simulink model "UGRP_Drone_Modeling4_with_motor_dynamics_v2_current_model"  (R2021b)
settings: Solver=FixedStepAuto  StartTime=0.0  StopTime=27  FixedStep=1/600
undefined symbols (not defined in the file or in its folder): sigbuilder_block
libraries: sim3dlib x1, uavsim3dlib x1
settings Model: Creator=user  LastModifiedBy=user
settings SolverCC: MaxConsecutiveMinStep=5  ShapePreserveControl=EnableAll  ZeroCrossAlgorithm=Adaptive
settings DebuggingCC: MaskedZcDiagnostic=none  IgnoredZcDiagnostic=none
settings SFSimCC: SimHardwareAcceleration=native  SimTargetLang=C++

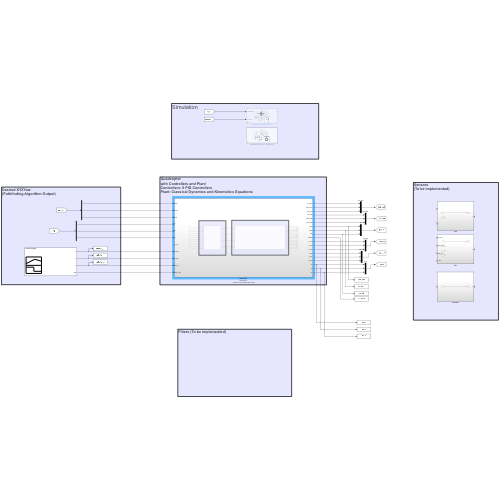
[thumbnail: Simulink's stored preview of the top-level diagram]
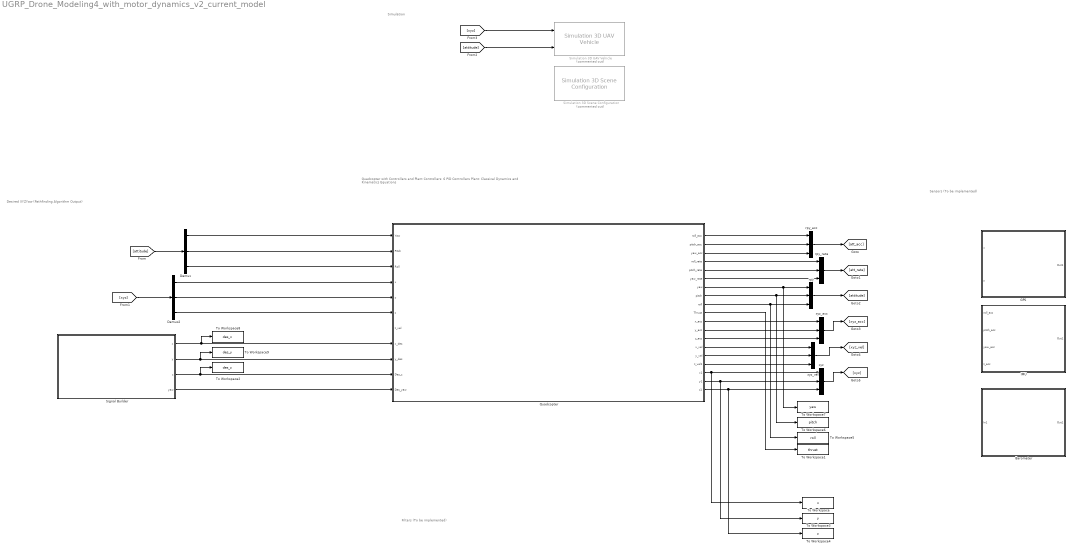
== system UGRP_Drone_Modeling4_with_motor_dynamics_v2_current_model ==
  note: Filters (To be implemented)
  note: Sensors
      | (To be implemented)
  note: Desired XYZYaw
      | (Pathfinding Algorithm Output)
  note: Quadcopter
      | with Controllers and Plant
      | Controllers: 6 PID Controllers
      | Plant: Classical Dynamics and Kinematics Equations
  note: Simulation
  Barometer : Subsystem
  Demux : Demux  Outputs=3
  Demux2 : Demux  Outputs=3
  GPS : Subsystem
  IMU : Subsystem
  Quadcopter : Subsystem  Description=Quadcopter including controllers and plant
      settings: AttributesFormatString=|
      | Quadcopter
      | - Controller and Quadcopter Plant
  Signal Builder : Subsystem  Tag=STV Subsys  LoadFcn=sigbuilder_block('load');  StartFcn=sigbuilder_block('start');  StopFcn=sigbuilder_block('stop');  ClipboardFcn=sigbuilder_block('clipboard');  mask(Sigbuilder block){tuvar=[0:10]}
      mask help: Simulink:masks:SigbuilderBlock_MD
      mask init:
      | if ~strcmp(get_param(bdroot(gcbh),'SimulationStatus'),'stopped') tuvar = sigbuilder_block('maskInit'); end
      settings: CopyFcn=sigbuilder_block('copy');  DeleteFcn=sigbuilder_block('delete');  ModelCloseFcn=sigbuilder_block('modelClose');  PreSaveFcn=sigbuilder_block('preSave');  PauseFcn=sigbuilder_block('pause');  ContinueFcn=sigbuilder_block('continue');  NameChangeFcn=sigbuilder_block('namechange');  OpenFcn=sigbuilder_block('open',[304.5 213 821.25 385.5 ]);  CloseFcn=sigbuilder_block('close');
      mask Display: plot(0, 0, 100, 100,[2, 2, 32, 32, 2], [68, 8, 8, 68, 68],[32, 2], [38, 38], [32, 19, 2],[53, 60, 44], [32, 17, 17, 2],[16, 16, 31, 31]);txt = getActiveGroup(gcbh);text(2, 100, txt,'verticalAlignment', 'top');
  Simulation 3D Scene Configuration : sim3dlib/Simulation 3D Scene Configuration  Priority=0  Commented=on  ProjectFormat_internal=Default Scenes  ProjectFormat=Default Scenes  SceneDesc=US city block  ProjectName=C:\Program Files\MATLAB\R2021b\toolbox\shared\sim3d_projects\automotive_project\UE4\WindowsNoEditor\VehicleSimulation.exe  ScenePath=/Game/Maps/USCityBlock  vehTagList={'Scene Origin';'SimulinkVehicle1'}  vehTag=SimulinkVehicle1  OpVisEn=off  Ts=1/60  EnableWindow=on  EnableWeather=off  SunAltitude=40.0  SunAzimuth=90  clouds=10  wind=1  fog=0  rain=0  sensorTag=MainCamera1  sensorId=1  sensorName=MainCamera1  mountLoc=Origin  offsetFlag=off  tmountOffset=[0, 0, 0]  rmountOffset=[0, 0, 0]  HorizontalResolution=1280  VerticalResolution=720  HorizontalFOV=60  mountPoint=[0 0 0]  mountOrientation=[0 0 0]  aMode=4  ID=1
      settings: SourceProductBaseCode=AE,DR,UV,VE
  Simulation 3D UAV Vehicle : uavsim3dlib/Simulation 3D UAV Vehicle  Priority=-1  Commented=on  Mesh=Quadrotor  MeshPath=/MathWorksUAVContent/UAVs/HexaRotorUAV/HexaRotor.HexaRotor  Color=Black  ActorName=SimulinkVehicle1  InitialTranslation=[0 0 0]  InitialRotation=[0 0 0]  SampleTime=-1  ActorType=SimulinkVehicle  ID=1  aMode=4  ActorTag=SimulinkVehicle1
      settings: SourceProductBaseCode=UV
  To Workspace : ToWorkspace  VariableName=x  SaveFormat=Timeseries  SampleTime=-1
  To Workspace1 : ToWorkspace  VariableName=thrust  SaveFormat=Timeseries  SampleTime=-1
  To Workspace2 : ToWorkspace  VariableName=des_z  SaveFormat=Timeseries  SampleTime=-1
  To Workspace3 : ToWorkspace  VariableName=y  SaveFormat=Timeseries  SampleTime=-1
  To Workspace4 : ToWorkspace  VariableName=z  SaveFormat=Timeseries  SampleTime=-1
  To Workspace5 : ToWorkspace  VariableName=roll  SaveFormat=Timeseries  SampleTime=-1
  To Workspace6 : ToWorkspace  VariableName=pitch  SaveFormat=Timeseries  SampleTime=-1
  To Workspace7 : ToWorkspace  VariableName=yaw  SaveFormat=Timeseries  SampleTime=-1
  To Workspace8 : ToWorkspace  VariableName=des_x  SaveFormat=Timeseries  SampleTime=-1
  To Workspace9 : ToWorkspace  VariableName=des_y  SaveFormat=Timeseries  SampleTime=-1
  rpy : Mux  Inputs=3
  rpy_acc : Mux  Inputs=3
  rpy_rate : Mux  Inputs=3
  xyz : Mux  Inputs=3
  xyz_acc : Mux  Inputs=3
  xyz_vel : Mux  Inputs=3
  wires:
  Signal Builder/3(z) -> Quadcopter/10(Des_z), To Workspace2/1
  xyz/1 -> [xyz]
  rpy/1 -> [attitude]
  rpy_acc/1 -> [att_acc]
  rpy_rate/1 -> [att_rate]
  xyz_acc/1 -> [xyz_acc]
  xyz_vel/1 -> [xyz_vel]
  [xyz] -> Demux2/1
  [attitude] -> Demux/1
  Quadcopter/7(yaw) -> rpy/1, To Workspace7/1
  Quadcopter/9(roll) -> rpy/3, To Workspace5/1
  Quadcopter/8(pitch) -> To Workspace6/1, rpy/2
  Demux/1 -> Quadcopter/1(Yaw)
  Demux/2 -> Quadcopter/2(Pitch)
  Demux/3 -> Quadcopter/3(Roll)
  Demux2/1 -> Quadcopter/4(x)
  Demux2/2 -> Quadcopter/5(y)
  Demux2/3 -> Quadcopter/6(z)
  Signal Builder/4(yaw) -> Quadcopter/11(Des_yaw)
  Quadcopter/1(roll_acc) -> rpy_acc/1
  Quadcopter/2(pitch_acc) -> rpy_acc/2
  Quadcopter/3(yaw_acc) -> rpy_acc/3
  Quadcopter/4(roll_rate) -> rpy_rate/1
  Quadcopter/5(pitch_rate) -> rpy_rate/2
  Quadcopter/6(yaw_rate) -> rpy_rate/3
  Quadcopter/11(x_acc) -> xyz_acc/1
  Quadcopter/12(y_acc) -> xyz_acc/2
  Quadcopter/13(z_acc) -> xyz_acc/3
  Quadcopter/14(x_vel) -> xyz_vel/1
  Quadcopter/15(y_vel) -> xyz_vel/2
  Quadcopter/16(z_vel1) -> xyz_vel/3
  Quadcopter/17(x1) -> xyz/1, To Workspace/1
  Quadcopter/18(y1) -> xyz/2, To Workspace3/1
  Quadcopter/19(z1) -> xyz/3, To Workspace4/1
  Quadcopter/10(Thrust) -> To Workspace1/1
  [xyz] -> Simulation 3D UAV Vehicle/1
  [attitude] -> Simulation 3D UAV Vehicle/2
  Signal Builder/1(x) -> Quadcopter/8(x_des), To Workspace8/1
  Signal Builder/2(y) -> Quadcopter/9(y_des), To Workspace9/1

== system UGRP_Drone_Modeling4_with_motor_dynamics_v2_current_model/Barometer ==
  In1 : Inport
  Out1 : Outport
  wires:
  In1/1 -> Out1/1

== system UGRP_Drone_Modeling4_with_motor_dynamics_v2_current_model/GPS ==
  x : Inport
  y : Inport  Port=2
  Out1 : Outport
  wires:
  x/1 -> Out1/1

== system UGRP_Drone_Modeling4_with_motor_dynamics_v2_current_model/IMU ==
  roll_acc : Inport
  pitch_acc : Inport  Port=2
  yaw_acc : Inport  Port=3
  z_acc : Inport  Port=4
  Out1 : Outport
  wires:
  roll_acc/1 -> Out1/1

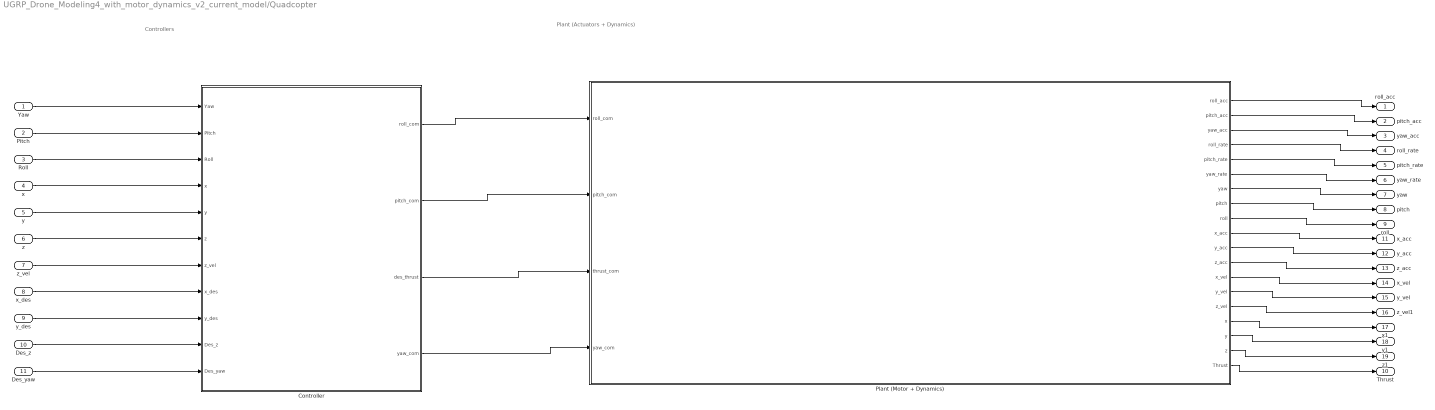
== system UGRP_Drone_Modeling4_with_motor_dynamics_v2_current_model/Quadcopter ==
  note: Plant (Actuators + Dynamics)
  note: Controllers
  Yaw : Inport
  Pitch : Inport  Port=2
  Roll : Inport  Port=3
  x : Inport  Port=4
  y : Inport  Port=5
  z : Inport  Port=6
  z_vel : Inport  Port=7
  x_des : Inport  Port=8
  y_des : Inport  Port=9
  Des_z : Inport  Port=10
  Des_yaw : Inport  Port=11
  Controller : Subsystem
  Plant (Motor + Dynamics) : Subsystem
  roll_acc : Outport
  pitch_acc : Outport  Port=2
  yaw_acc : Outport  Port=3
  roll_rate : Outport  Port=4
  pitch_rate : Outport  Port=5
  yaw_rate : Outport  Port=6
  yaw : Outport  Port=7
  pitch : Outport  Port=8
  roll : Outport  Port=9
  Thrust : Outport  Port=10
  x_acc : Outport  Port=11
  y_acc : Outport  Port=12
  z_acc : Outport  Port=13
  x_vel : Outport  Port=14
  y_vel : Outport  Port=15
  z_vel1 : Outport  Port=16
  x1 : Outport  Port=17
  y1 : Outport  Port=18
  z1 : Outport  Port=19
  wires:
  Plant (Motor + Dynamics)/14(y_vel) -> y_vel/1
  Plant (Motor + Dynamics)/9(roll) -> roll/1
  x_des/1 -> Controller/8(x_des)
  Controller/1(roll_com) -> Plant (Motor + Dynamics)/1(roll_com)
  Plant (Motor + Dynamics)/6(yaw_rate) -> yaw_rate/1
  Plant (Motor + Dynamics)/7(yaw) -> yaw/1
  Plant (Motor + Dynamics)/17(y) -> y1/1
  Plant (Motor + Dynamics)/18(z) -> z1/1
  Controller/2(pitch_com) -> Plant (Motor + Dynamics)/2(pitch_com)
  Plant (Motor + Dynamics)/5(pitch_rate) -> pitch_rate/1
  Plant (Motor + Dynamics)/10(x_acc) -> x_acc/1
  Des_yaw/1 -> Controller/11(Des_yaw)
  Controller/3(des_thrust) -> Plant (Motor + Dynamics)/3(thrust_com)
  Plant (Motor + Dynamics)/8(pitch) -> pitch/1
  Controller/4(yaw_com) -> Plant (Motor + Dynamics)/4(yaw_com)
  Plant (Motor + Dynamics)/13(x_vel) -> x_vel/1
  y/1 -> Controller/5(y)
  Plant (Motor + Dynamics)/1(roll_acc) -> roll_acc/1
  Des_z/1 -> Controller/10(Des_z)
  Plant (Motor + Dynamics)/19(Thrust) -> Thrust/1
  x/1 -> Controller/4(x)
  Plant (Motor + Dynamics)/3(yaw_acc) -> yaw_acc/1
  Plant (Motor + Dynamics)/12(z_acc) -> z_acc/1
  Plant (Motor + Dynamics)/11(y_acc) -> y_acc/1
  Roll/1 -> Controller/3(Roll)
  Plant (Motor + Dynamics)/15(z_vel) -> z_vel1/1
  z_vel/1 -> Controller/7(z_vel)
  Plant (Motor + Dynamics)/16(x) -> x1/1
  y_des/1 -> Controller/9(y_des)
  Yaw/1 -> Controller/1(Yaw)
  Plant (Motor + Dynamics)/2(pitch_acc) -> pitch_acc/1
  z/1 -> Controller/6(z)
  Pitch/1 -> Controller/2(Pitch)
  Plant (Motor + Dynamics)/4(roll_rate) -> roll_rate/1

== system UGRP_Drone_Modeling4_with_motor_dynamics_v2_current_model/Signal Builder ==
  Demux : Demux  Tag=STV Demux
      settings: DisplayOption=none
  FromWs : FromWorkspace  Tag=STV FromWs  VariableName=tuvar
      SigBuilderData=|
      | common.afterFinalStr = 'Extrapolate'
      | common.sampleTime = 0
      | dataSet.timeRange = [0 25]
      | dataSet.name = 'Desired xyzyaw'
      | sbobj.Groups.Name = 'Desired xyzyaw'
      | sbobj.Groups.Signals(1).Name = 'x'
      | sbobj.Groups.Signals(1).XData = [0 12 12 20 20 25]
      | sbobj.Groups.Signals(1).YData = [0 0 2 2 0 0]
      | sbobj.Groups.Signals(2).Name = 'y'
      | sbobj.Groups.Signals(2).XData = [0 3.99 12 12 20 20 25]
      | sbobj.Groups.Signals(2).YData = [0 0 0 -2 -2 0 0]
      | sbobj.Groups.Signals(3).Name = 'z'
      | sbobj.Groups.Signals(3).XData = [0 25]
      | sbobj.Groups.Signals(3).YData = [3 3]
      | sbobj.Groups.Signals(4).Name = 'yaw'
      | sbobj.Groups.Signals(4).XData = [0 5 8 25]
      | sbobj.Groups.Signals(4).YData = [0 0 0 0]
      | sbobj.Groups.TimeRange = [0 25]
  x : Outport  Tag=STV Outport
  y : Outport  Tag=STV Outport  Port=2
  z : Outport  Tag=STV Outport  Port=3
  yaw : Outport  Tag=STV Outport  Port=4
  wires:
  FromWs/1 -> Demux/1
  Demux/1 -> x/1
  Demux/2 -> y/1
  Demux/3 -> z/1
  Demux/4 -> yaw/1

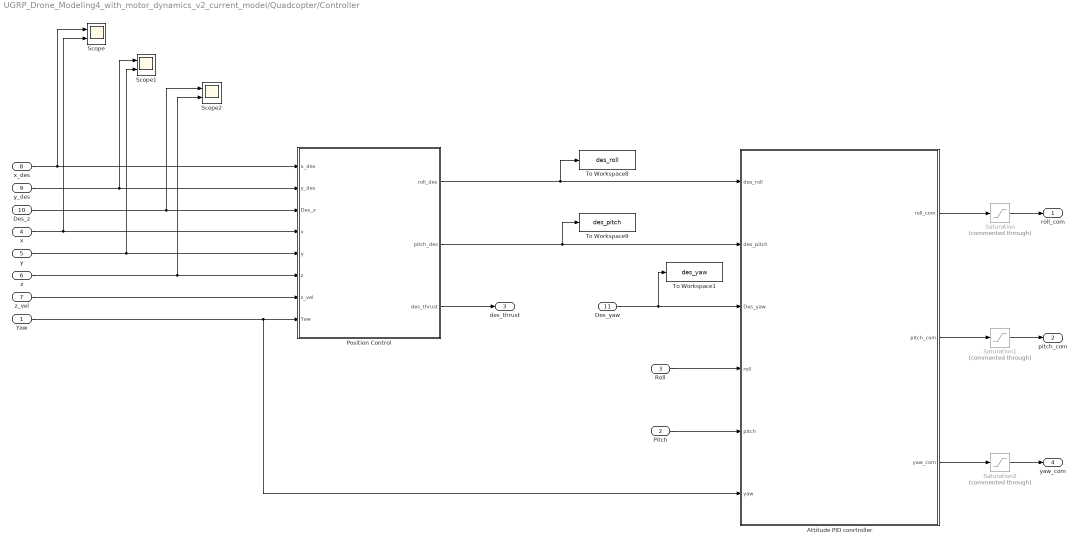
== system UGRP_Drone_Modeling4_with_motor_dynamics_v2_current_model/Quadcopter/Controller ==
  Yaw : Inport
  Pitch : Inport  Port=2
  Roll : Inport  Port=3
  x : Inport  Port=4
  y : Inport  Port=5
  z : Inport  Port=6
  z_vel : Inport  Port=7
  x_des : Inport  Port=8
  y_des : Inport  Port=9
  Des_z : Inport  Port=10
  Des_yaw : Inport  Port=11
  Attitude PID conrtroller : Subsystem
  Position Control : Subsystem
  Saturation : Saturate  Commented=through  UpperLimit=4  LowerLimit=-4
  Saturation1 : Saturate  Commented=through  UpperLimit=1  LowerLimit=-1
  Saturation2 : Saturate  Commented=through  UpperLimit=1  LowerLimit=-1
  Scope : Scope  NumInputPorts=2
  Scope1 : Scope  NumInputPorts=2
  Scope2 : Scope  NumInputPorts=2
  To Workspace1 : ToWorkspace  VariableName=des_yaw  SaveFormat=Timeseries  SampleTime=-1
  To Workspace8 : ToWorkspace  VariableName=des_roll  SaveFormat=Timeseries  SampleTime=-1
  To Workspace9 : ToWorkspace  VariableName=des_pitch  SaveFormat=Timeseries  SampleTime=-1
  roll_com : Outport
  pitch_com : Outport  Port=2
  des_thrust : Outport  Port=3
  yaw_com : Outport  Port=4
  wires:
  z_vel/1 -> Position Control/7(z_vel)
  Attitude PID conrtroller/2(pitch_com) -> Saturation1/1
  Position Control/3(des_thrust) -> des_thrust/1
  y/1 -> Scope1/2, Position Control/5(y)
  Attitude PID conrtroller/3(yaw_com) -> Saturation2/1
  Attitude PID conrtroller/1(roll_com) -> Saturation/1
  Des_yaw/1 -> Attitude PID conrtroller/3(Des_yaw), To Workspace1/1
  x_des/1 -> Position Control/1(x_des), Scope/1
  z/1 -> Position Control/6(z), Scope2/2
  Des_z/1 -> Position Control/3(Des_z), Scope2/1
  y_des/1 -> Scope1/1, Position Control/2(y_des)
  Yaw/1 -> Attitude PID conrtroller/6(yaw), Position Control/8(Yaw)
  x/1 -> Position Control/4(x), Scope/2
  Position Control/2(pitch_des) -> To Workspace9/1, Attitude PID conrtroller/2(des_pitch)
  Position Control/1(roll_des) -> To Workspace8/1, Attitude PID conrtroller/1(des_roll)
  Roll/1 -> Attitude PID conrtroller/4(roll)
  Pitch/1 -> Attitude PID conrtroller/5(pitch)
  Saturation/1 -> roll_com/1
  Saturation1/1 -> pitch_com/1
  Saturation2/1 -> yaw_com/1

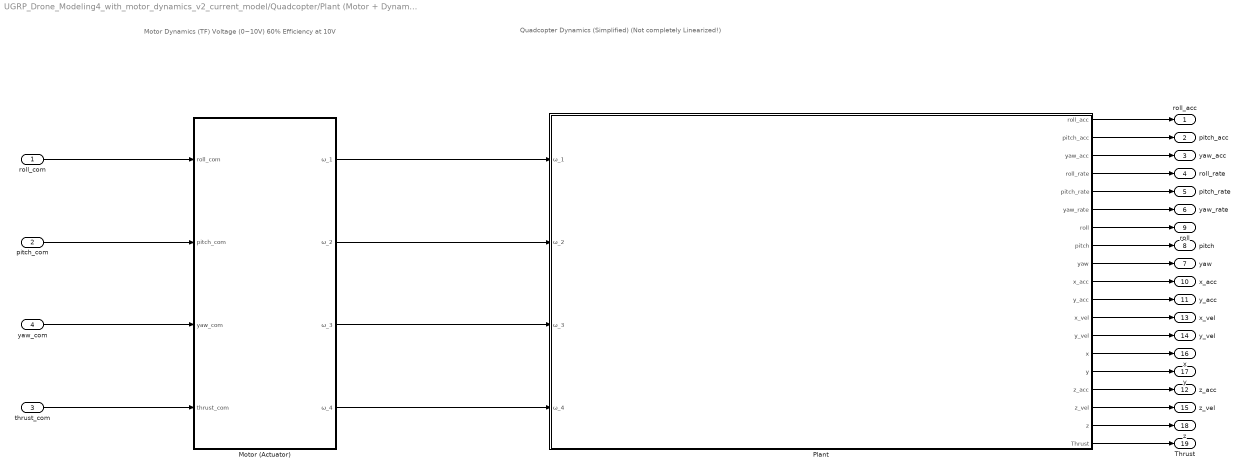
== system UGRP_Drone_Modeling4_with_motor_dynamics_v2_current_model/Quadcopter/Plant (Motor + Dynamics) ==
  note: Quadcopter Dynamics  (Simplified)
      | (Not completely Linearized!)
  note: Motor Dynamics (TF)
      | Voltage (0~10V)
      | 60% Efficiency at 10V
  roll_com : Inport
  pitch_com : Inport  Port=2
  thrust_com : Inport  Port=3
  yaw_com : Inport  Port=4
  Motor (Actuator) : Subsystem
  Plant : Subsystem
  roll_acc : Outport
  pitch_acc : Outport  Port=2
  yaw_acc : Outport  Port=3
  roll_rate : Outport  Port=4
  pitch_rate : Outport  Port=5
  yaw_rate : Outport  Port=6
  yaw : Outport  Port=7
  pitch : Outport  Port=8
  roll : Outport  Port=9
  x_acc : Outport  Port=10
  y_acc : Outport  Port=11
  z_acc : Outport  Port=12
  x_vel : Outport  Port=13
  y_vel : Outport  Port=14
  z_vel : Outport  Port=15
  x : Outport  Port=16
  y : Outport  Port=17
  z : Outport  Port=18
  Thrust : Outport  Port=19
  wires:
  Plant/9(yaw) -> yaw/1
  Motor (Actuator)/1(ω_1) -> Plant/1(ω_1)
  Plant/2(pitch_acc) -> pitch_acc/1
  Motor (Actuator)/2(ω_2) -> Plant/2(ω_2)
  Plant/7(roll) -> roll/1
  Motor (Actuator)/4(ω_4) -> Plant/4(ω_4)
  Plant/6(yaw_rate) -> yaw_rate/1
  Plant/8(pitch) -> pitch/1
  Plant/5(pitch_rate) -> pitch_rate/1
  Motor (Actuator)/3(ω_3) -> Plant/3(ω_3)
  Plant/12(x_vel) -> x_vel/1
  Plant/11(y_acc) -> y_acc/1
  Plant/13(y_vel) -> y_vel/1
  Plant/4(roll_rate) -> roll_rate/1
  Plant/1(roll_acc) -> roll_acc/1
  roll_com/1 -> Motor (Actuator)/1(roll_com)
  Plant/3(yaw_acc) -> yaw_acc/1
  Plant/10(x_acc) -> x_acc/1
  pitch_com/1 -> Motor (Actuator)/2(pitch_com)
  Plant/14(x) -> x/1
  Plant/16(z_acc) -> z_acc/1
  Plant/19(Thrust) -> Thrust/1
  Plant/15(y) -> y/1
  Plant/17(z_vel) -> z_vel/1
  Plant/18(z) -> z/1
  yaw_com/1 -> Motor (Actuator)/3(yaw_com)
  thrust_com/1 -> Motor (Actuator)/4(thrust_com)

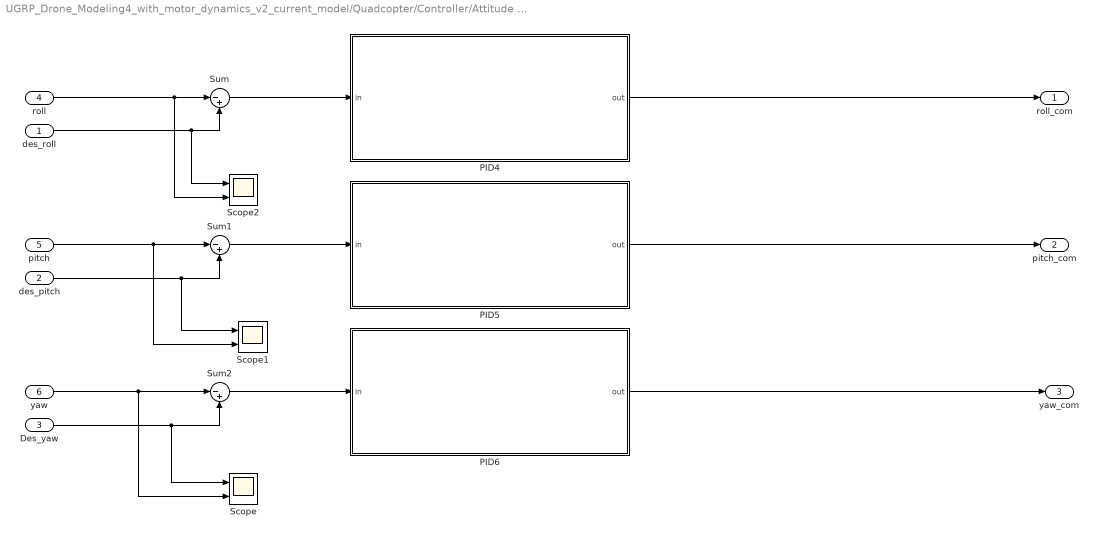
== system UGRP_Drone_Modeling4_with_motor_dynamics_v2_current_model/Quadcopter/Controller/Attitude PID conrtroller ==
  des_roll : Inport
  des_pitch : Inport  Port=2
  Des_yaw : Inport  Port=3
  roll : Inport  Port=4
  pitch : Inport  Port=5
  yaw : Inport  Port=6
  PID4 : Subsystem
  PID5 : Subsystem
  PID6 : Subsystem
  Scope : Scope  NumInputPorts=2
  Scope1 : Scope  NumInputPorts=2
  Scope2 : Scope  NumInputPorts=2
  Sum : Sum  Inputs=|-+
  Sum1 : Sum  Inputs=|-+
  Sum2 : Sum  Inputs=|-+
  roll_com : Outport
  pitch_com : Outport  Port=2
  yaw_com : Outport  Port=3
  wires:
  des_roll/1 -> Scope2/1, Sum/2
  Des_yaw/1 -> Scope/1, Sum2/2
  yaw/1 -> Scope/2, Sum2/1
  Sum/1 -> PID4/1(in)
  Sum2/1 -> PID6/1(in)
  Sum1/1 -> PID5/1(in)
  pitch/1 -> Scope1/2, Sum1/1
  des_pitch/1 -> Scope1/1, Sum1/2
  roll/1 -> Scope2/2, Sum/1
  PID4/1(out) -> roll_com/1
  PID5/1(out) -> pitch_com/1
  PID6/1(out) -> yaw_com/1

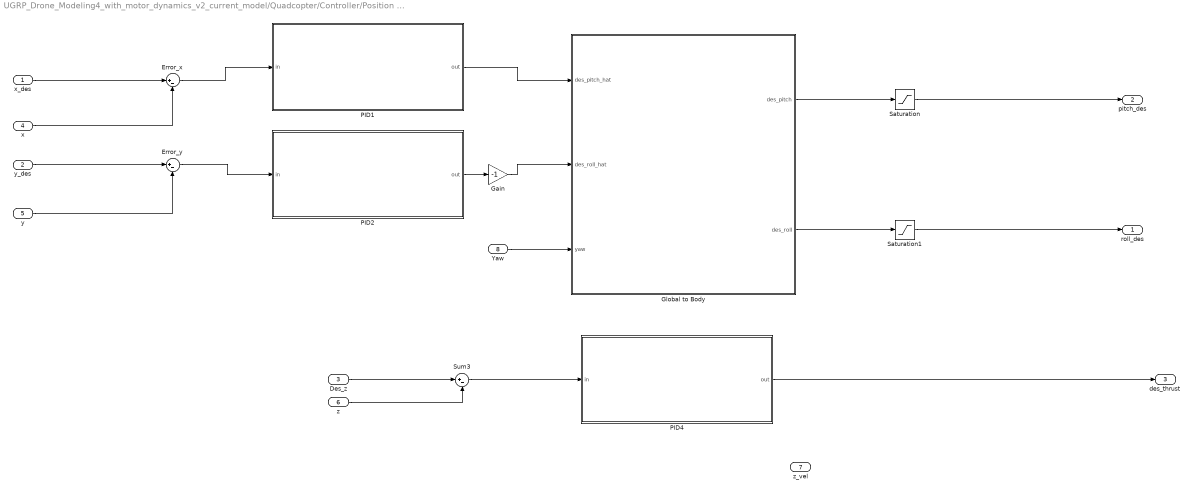
== system UGRP_Drone_Modeling4_with_motor_dynamics_v2_current_model/Quadcopter/Controller/Position Control ==
  x_des : Inport
  y_des : Inport  Port=2
  Des_z : Inport  Port=3
  x : Inport  Port=4
  y : Inport  Port=5
  z : Inport  Port=6
  z_vel : Inport  Port=7
  Yaw : Inport  Port=8
  Error_x : Sum  Inputs=|+-
  Error_y : Sum  Inputs=|+-
  Gain : Gain  Gain=-1
  Global to Body : Subsystem
  PID1 : Subsystem
  PID2 : Subsystem
  PID4 : Subsystem
  Saturation : Saturate  UpperLimit=10*pi/180  LowerLimit=-10*pi/180
  Saturation1 : Saturate  UpperLimit=10*pi/180  LowerLimit=-10*pi/180
  Sum3 : Sum  Inputs=|+-
  roll_des : Outport
  pitch_des : Outport  Port=2
  des_thrust : Outport  Port=3
  wires:
  x_des/1 -> Error_x/1
  x/1 -> Error_x/2
  y_des/1 -> Error_y/1
  y/1 -> Error_y/2
  Des_z/1 -> Sum3/1
  Yaw/1 -> Global to Body/3(yaw)
  Error_y/1 -> PID2/1(in)
  Error_x/1 -> PID1/1(in)
  Global to Body/2(des_roll) -> Saturation1/1
  z/1 -> Sum3/2
  Global to Body/1(des_pitch) -> Saturation/1
  PID1/1(out) -> Global to Body/1(des_pitch_hat)
  PID2/1(out) -> Gain/1
  Gain/1 -> Global to Body/2(des_roll_hat)
  Saturation1/1 -> roll_des/1
  Saturation/1 -> pitch_des/1
  Sum3/1 -> PID4/1(in)
  PID4/1(out) -> des_thrust/1

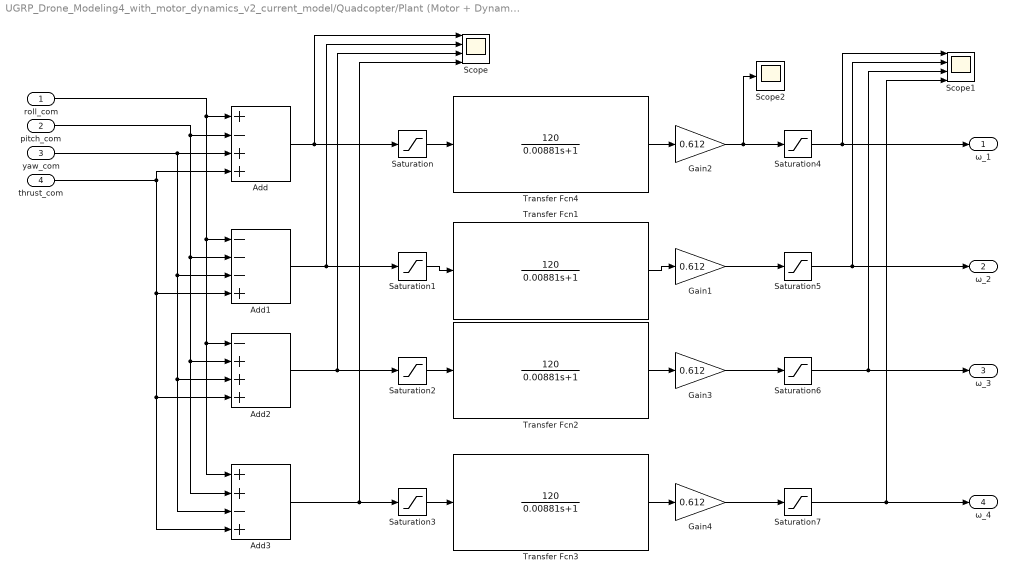
== system UGRP_Drone_Modeling4_with_motor_dynamics_v2_current_model/Quadcopter/Plant (Motor + Dynamics)/Motor (Actuator) ==
  roll_com : Inport
  pitch_com : Inport  Port=2
  yaw_com : Inport  Port=3
  thrust_com : Inport  Port=4
  Add : Sum  Inputs=+-++
  Add1 : Sum  Inputs=---+
  Add2 : Sum  Inputs=-+++
  Add3 : Sum  Inputs=++-+
  Gain{1..4} (4 alike) : Gain  Gain=0.612
  Saturation{,1..3} (4 alike) : Saturate  UpperLimit=10  LowerLimit=0
  Saturation{4..7} (4 alike) : Saturate  UpperLimit=1040  LowerLimit=0
  Scope : Scope  NumInputPorts=4
  Scope1 : Scope  NumInputPorts=4
  Scope2 : Scope
  Transfer Fcn{1..4} (4 alike) : TransferFcn  Numerator=[120]  Denominator=[0.00881 1]
  ω_1 : Outport
  ω_2 : Outport  Port=2
  ω_3 : Outport  Port=3
  ω_4 : Outport  Port=4
  wires:
  roll_com/1 -> Add3/1, Add2/1, Add1/1, Add/1
  pitch_com/1 -> Add3/2, Add2/2, Add1/2, Add/2
  yaw_com/1 -> Add3/3, Add2/3, Add1/3, Add/3
  thrust_com/1 -> Add/4, Add3/4, Add2/4, Add1/4
  Add/1 -> Saturation/1, Scope/1
  Add1/1 -> Saturation1/1, Scope/2
  Add2/1 -> Saturation2/1, Scope/3
  Add3/1 -> Scope/4, Saturation3/1
  Saturation/1 -> Transfer Fcn4/1
  Saturation2/1 -> Transfer Fcn2/1
  Saturation1/1 -> Transfer Fcn1/1
  Saturation3/1 -> Transfer Fcn3/1
  Saturation4/1 -> Scope1/1, ω_1/1
  Saturation5/1 -> Scope1/2, ω_2/1
  Saturation6/1 -> Scope1/3, ω_3/1
  Saturation7/1 -> Scope1/4, ω_4/1
  Transfer Fcn4/1 -> Gain2/1
  Gain2/1 -> Scope2/1, Saturation4/1
  Transfer Fcn1/1 -> Gain1/1
  Gain1/1 -> Saturation5/1
  Transfer Fcn2/1 -> Gain3/1
  Gain3/1 -> Saturation6/1
  Transfer Fcn3/1 -> Gain4/1
  Gain4/1 -> Saturation7/1

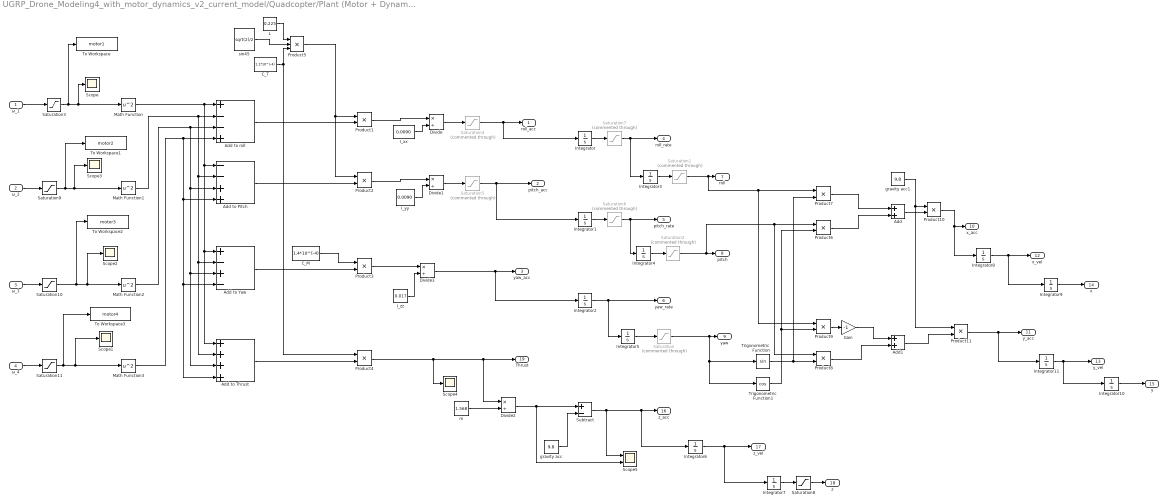
== system UGRP_Drone_Modeling4_with_motor_dynamics_v2_current_model/Quadcopter/Plant (Motor + Dynamics)/Plant ==
  ω_1 : Inport
  ω_2 : Inport  Port=2
  ω_3 : Inport  Port=3
  ω_4 : Inport  Port=4
  Add : Sum
  Add to Pitch : Sum  Inputs=--++  RndMeth=Round
  Add to Thrust : Sum  Inputs=++++  RndMeth=Round
  Add to Yaw : Sum  Inputs=+-+-  RndMeth=Round
  Add to roll : Sum  Inputs=+--+
  Add1 : Sum
  C_M : Constant  Value=1.4*10^(-4)
  C_T : Constant  Value=1.1*10^(-4)
  Divide{,1..3} (4 alike) : Product  Inputs=*/
  Gain : Gain  Gain=-1
  I_xx : Constant  Value=0.0090
  I_yy : Constant  Value=0.0090
  I_zz : Constant  Value=0.017
  Integrator{,1,6..11} (8 alike) : Integrator
  Integrator2 : Integrator  LimitOutput=on  UpperSaturationLimit=2*pi  LowerSaturationLimit=-2*pi  WrappedStateUpperValue=2*pi  WrappedStateLowerValue=-2*pi
  Integrator3 : Integrator  LimitOutput=on  UpperSaturationLimit=10*pi/180  LowerSaturationLimit=-10*pi/180  WrappedStateUpperValue=10*pi/180  WrappedStateLowerValue=-10*pi/180
  Integrator4 : Integrator  LimitOutput=on  UpperSaturationLimit=10*pi/180  LowerSaturationLimit=-10*pi/180  WrappedStateUpperValue=10*pi/180  WrappedStateLowerValue=-10*pi/180
  Integrator5 : Integrator  UpperSaturationLimit=pi  LowerSaturationLimit=-pi
  L : Constant  Value=0.225
  Math Function : Math  Operator=square  RndMeth=Round  SaturateOnIntegerOverflow=on
  Math Function1 : Math  Operator=square  SaturateOnIntegerOverflow=on
  Math Function2 : Math  Operator=square  SaturateOnIntegerOverflow=on
  Math Function3 : Math  Operator=square  SaturateOnIntegerOverflow=on
  Product{1..4,6..11} (10 alike) : Product
  Product5 : Product  Inputs=3
  Saturation : Saturate  Commented=through  UpperLimit=2*pi  LowerLimit=-2*pi
  Saturation1 : Saturate  Commented=through  UpperLimit=10*pi/180  LowerLimit=-10*pi/180
  Saturation{3,9..11} (4 alike) : Saturate  UpperLimit=1000  LowerLimit=0
  Saturation2 : Saturate  Commented=through  UpperLimit=10*pi/180  LowerLimit=-10*pi/180
  Saturation{4..7} (4 alike) : Saturate  Commented=through  UpperLimit=1  LowerLimit=-1
  Saturation8 : Saturate  UpperLimit=inf  LowerLimit=0
  Scope{,1..4} (5 alike) : Scope
  Scope5 : Scope  NumInputPorts=2
  Subtract : Sum  Inputs=+-
  To Workspace : ToWorkspace  VariableName=motor1  SaveFormat=Timeseries  SampleTime=-1
  To Workspace1 : ToWorkspace  VariableName=motor2  SaveFormat=Timeseries  SampleTime=-1
  To Workspace2 : ToWorkspace  VariableName=motor3  SaveFormat=Timeseries  SampleTime=-1
  To Workspace3 : ToWorkspace  VariableName=motor4  SaveFormat=Timeseries  SampleTime=-1
  Trigonometric Function : Trigonometry
  Trigonometric Function1 : Trigonometry  Operator=cos
  gravity acc : Constant  Value=9.8
  gravity acc1 : Constant  Value=9.8
  m : Constant  Value=1.568
  sin45 : Constant  Value=sqrt(2)/2
  roll_acc : Outport
  pitch_acc : Outport  Port=2
  yaw_acc : Outport  Port=3
  roll_rate : Outport  Port=4
  pitch_rate : Outport  Port=5
  yaw_rate : Outport  Port=6
  roll : Outport  Port=7
  pitch : Outport  Port=8
  yaw : Outport  Port=9
  x_acc : Outport  Port=10
  y_acc : Outport  Port=11
  x_vel : Outport  Port=12
  y_vel : Outport  Port=13
  x : Outport  Port=14
  y : Outport  Port=15
  z_acc : Outport  Port=16
  z_vel : Outport  Port=17
  z : Outport  Port=18
  Thrust : Outport  Port=19
  wires:
  Product5/1 -> Product2/1, Product1/1
  ω_1/1 -> Saturation3/1
  ω_3/1 -> Saturation10/1
  ω_4/1 -> Saturation11/1
  Math Function/1 -> Add to Thrust/1, Add to Yaw/1, Add to Pitch/1, Add to roll/1
  Math Function1/1 -> Add to Thrust/2, Add to Yaw/2, Add to Pitch/2, Add to roll/2
  Math Function2/1 -> Add to Thrust/3, Add to Yaw/3, Add to Pitch/3, Add to roll/3
  Math Function3/1 -> Add to Thrust/4, Add to Yaw/4, Add to Pitch/4, Add to roll/4
  Add to roll/1 -> Product1/2
  Add to Yaw/1 -> Product3/2
  Add to Thrust/1 -> Product4/2
  sin45/1 -> Product5/2
  L/1 -> Product5/1
  C_M/1 -> Product3/1
  Product1/1 -> Divide/1
  I_xx/1 -> Divide/2
  Product2/1 -> Divide1/1
  I_yy/1 -> Divide1/2
  Divide/1 -> Saturation4/1
  Integrator2/1 -> Integrator5/1, yaw_rate/1
  Integrator1/1 -> Saturation6/1
  Integrator/1 -> Saturation7/1
  m/1 -> Divide2/2
  gravity acc/1 -> Subtract/2
  Integrator4/1 -> Saturation2/1
  Integrator3/1 -> Saturation1/1
  Saturation1/1 -> Product9/1, Product7/1, roll/1
  Integrator6/1 -> Integrator7/1, z_vel/1
  Integrator7/1 -> Saturation8/1
  Integrator8/1 -> Integrator9/1, x_vel/1
  Integrator9/1 -> x/1
  Integrator10/1 -> y/1
  Integrator11/1 -> Integrator10/1, y_vel/1
  C_T/1 -> Product5/3, Product4/1
  Product3/1 -> Divide3/1
  I_zz/1 -> Divide3/2
  Saturation2/1 -> Product8/1, Product6/1, pitch/1
  Integrator5/1 -> Saturation/1
  Saturation/1 -> Trigonometric Function1/1, Trigonometric Function/1, yaw/1
  Add to Pitch/1 -> Product2/2
  Divide3/1 -> yaw_acc/1, Integrator2/1
  ω_2/1 -> Saturation9/1
  Saturation4/1 -> roll_acc/1, Integrator/1
  Divide1/1 -> Saturation5/1
  Saturation5/1 -> Integrator1/1, pitch_acc/1
  Saturation6/1 -> Integrator4/1, pitch_rate/1
  Saturation7/1 -> roll_rate/1, Integrator3/1
  Saturation8/1 -> z/1
  Divide2/1 -> Scope5/2, Subtract/1
  Product4/1 -> Scope4/1, Divide2/1, Thrust/1
  Subtract/1 -> Scope5/1, Integrator6/1, z_acc/1
  Saturation3/1 -> To Workspace/1, Scope/1, Math Function/1
  Saturation9/1 -> To Workspace1/1, Scope3/1, Math Function1/1
  Saturation10/1 -> To Workspace2/1, Scope2/1, Math Function2/1
  Trigonometric Function1/1 -> Product9/2, Product6/2
  Product7/1 -> Add/1
  Product6/1 -> Add/2
  Product9/1 -> Gain/1
  Gain/1 -> Add1/1
  Product8/1 -> Add1/2
  Trigonometric Function/1 -> Product7/2, Product8/2
  Add/1 -> Product10/2
  Product10/1 -> Integrator8/1, x_acc/1
  gravity acc1/1 -> Product11/1, Product10/1
  Add1/1 -> Product11/2
  Product11/1 -> Integrator11/1, y_acc/1
  Saturation11/1 -> To Workspace3/1, Scope1/1, Math Function3/1

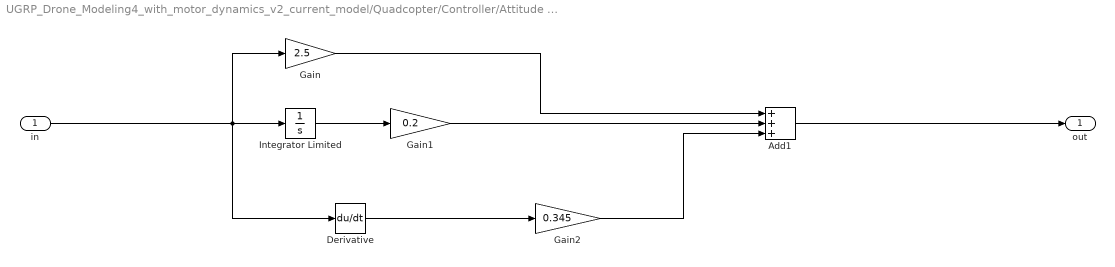
== system UGRP_Drone_Modeling4_with_motor_dynamics_v2_current_model/Quadcopter/Controller/Attitude PID conrtroller/PID4 ==
  in : Inport
  Add1 : Sum  Inputs=+++
  Derivative : Derivative
  Gain : Gain  Gain=2.5
  Gain1 : Gain  Gain=0.2
  Gain2 : Gain  Gain=0.345
  Integrator Limited : Integrator  LimitOutput=on  UpperSaturationLimit=10  LowerSaturationLimit=-10
  out : Outport
  wires:
  Integrator Limited/1 -> Gain1/1
  Gain/1 -> Add1/1
  Gain1/1 -> Add1/2
  Derivative/1 -> Gain2/1
  Gain2/1 -> Add1/3
  Add1/1 -> out/1
  in/1 -> Derivative/1, Gain/1, Integrator Limited/1

== system UGRP_Drone_Modeling4_with_motor_dynamics_v2_current_model/Quadcopter/Controller/Attitude PID conrtroller/PID5 ==
  in : Inport
  Add1 : Sum  Inputs=+++
  Derivative : Derivative
  Gain : Gain  Gain=2.5
  Gain1 : Gain  Gain=0.2
  Gain2 : Gain  Gain=0.345
  Integrator Limited : Integrator  LimitOutput=on  UpperSaturationLimit=10  LowerSaturationLimit=-10
  out : Outport
  wires:
  Integrator Limited/1 -> Gain1/1
  Gain/1 -> Add1/1
  Gain1/1 -> Add1/2
  Derivative/1 -> Gain2/1
  Gain2/1 -> Add1/3
  Add1/1 -> out/1
  in/1 -> Derivative/1, Gain/1, Integrator Limited/1

== system UGRP_Drone_Modeling4_with_motor_dynamics_v2_current_model/Quadcopter/Controller/Attitude PID conrtroller/PID6 ==
  in : Inport
  Add1 : Sum  Inputs=+++
  Derivative : Derivative
  Gain : Gain  Gain=0.09
  Gain1 : Gain  Gain=0
  Gain2 : Gain  Gain=0.06
  Integrator Limited : Integrator  LimitOutput=on  UpperSaturationLimit=10  LowerSaturationLimit=-10
  out : Outport
  wires:
  Integrator Limited/1 -> Gain1/1
  Gain/1 -> Add1/1
  in/1 -> Derivative/1, Gain/1, Integrator Limited/1
  Gain1/1 -> Add1/2
  Derivative/1 -> Gain2/1
  Gain2/1 -> Add1/3
  Add1/1 -> out/1

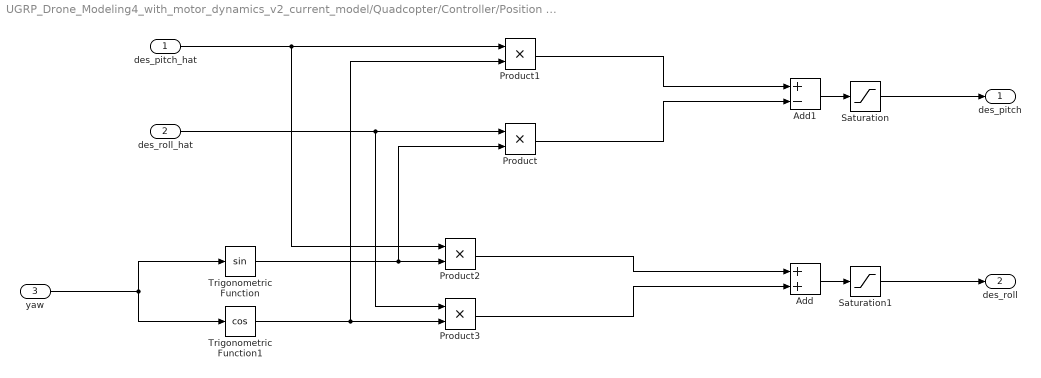
== system UGRP_Drone_Modeling4_with_motor_dynamics_v2_current_model/Quadcopter/Controller/Position Control/Global to Body ==
  des_pitch_hat : Inport
  des_roll_hat : Inport  Port=2
  yaw : Inport  Port=3
  Add : Sum
  Add1 : Sum  Inputs=+-
  Product{,1..3} (4 alike) : Product
  Saturation : Saturate  UpperLimit=10*pi/180  LowerLimit=-10*pi/180
  Saturation1 : Saturate  UpperLimit=10*pi/180  LowerLimit=-10*pi/180
  Trigonometric Function : Trigonometry
  Trigonometric Function1 : Trigonometry  Operator=cos
  des_pitch : Outport
  des_roll : Outport  Port=2
  wires:
  yaw/1 -> Trigonometric Function/1, Trigonometric Function1/1
  Add/1 -> Saturation1/1
  Add1/1 -> Saturation/1
  Saturation1/1 -> des_roll/1
  des_pitch_hat/1 -> Product2/1, Product1/1
  Product1/1 -> Add1/1
  Trigonometric Function1/1 -> Product3/2, Product1/2
  des_roll_hat/1 -> Product3/1, Product/1
  Trigonometric Function/1 -> Product2/2, Product/2
  Product/1 -> Add1/2
  Product2/1 -> Add/1
  Product3/1 -> Add/2
  Saturation/1 -> des_pitch/1

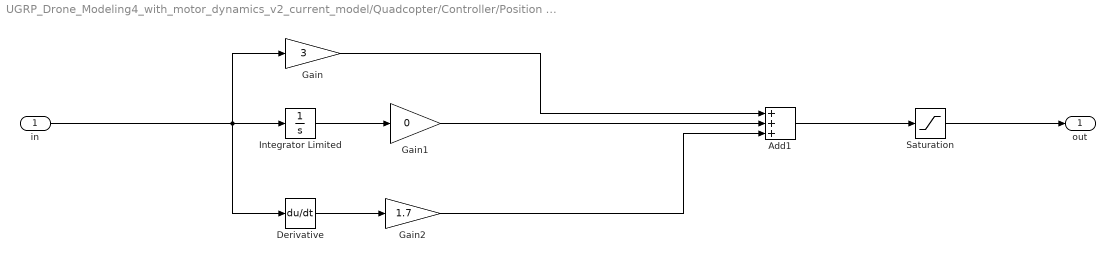
== system UGRP_Drone_Modeling4_with_motor_dynamics_v2_current_model/Quadcopter/Controller/Position Control/PID1 ==
  in : Inport
  Add1 : Sum  Inputs=+++
  Derivative : Derivative
  Gain : Gain  Gain=3
  Gain1 : Gain  Gain=0
  Gain2 : Gain  Gain=1.7
  Integrator Limited : Integrator  LimitOutput=on  UpperSaturationLimit=20  LowerSaturationLimit=-20
  Saturation : Saturate  UpperLimit=10*pi/180  LowerLimit=-10*pi/180
  out : Outport
  wires:
  Integrator Limited/1 -> Gain1/1
  in/1 -> Derivative/1, Gain/1, Integrator Limited/1
  Gain/1 -> Add1/1
  Gain1/1 -> Add1/2
  Derivative/1 -> Gain2/1
  Gain2/1 -> Add1/3
  Add1/1 -> Saturation/1
  Saturation/1 -> out/1

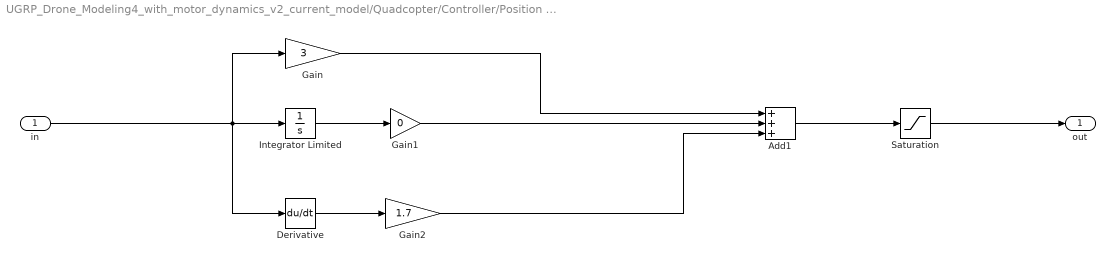
== system UGRP_Drone_Modeling4_with_motor_dynamics_v2_current_model/Quadcopter/Controller/Position Control/PID2 ==
  in : Inport
  Add1 : Sum  Inputs=+++
  Derivative : Derivative
  Gain : Gain  Gain=3
  Gain1 : Gain  Gain=0
  Gain2 : Gain  Gain=1.7
  Integrator Limited : Integrator  LimitOutput=on  UpperSaturationLimit=10  LowerSaturationLimit=-10
  Saturation : Saturate  UpperLimit=10*pi/180  LowerLimit=-10*pi/180
  out : Outport
  wires:
  Integrator Limited/1 -> Gain1/1
  in/1 -> Derivative/1, Gain/1, Integrator Limited/1
  Gain/1 -> Add1/1
  Gain1/1 -> Add1/2
  Derivative/1 -> Gain2/1
  Gain2/1 -> Add1/3
  Add1/1 -> Saturation/1
  Saturation/1 -> out/1

== system UGRP_Drone_Modeling4_with_motor_dynamics_v2_current_model/Quadcopter/Controller/Position Control/PID4 ==
  in : Inport
  Add1 : Sum  Inputs=+++
  Derivative : Derivative
  Gain : Gain  Gain=4.5
  Gain1 : Gain  Gain=2
  Gain2 : Gain  Gain=1.7
  Integrator Limited : Integrator  LimitOutput=on  UpperSaturationLimit=100  LowerSaturationLimit=-100
  out : Outport
  wires:
  Integrator Limited/1 -> Gain1/1
  Gain/1 -> Add1/1
  in/1 -> Derivative/1, Gain/1, Integrator Limited/1
  Gain1/1 -> Add1/2
  Gain2/1 -> Add1/3
  Add1/1 -> out/1
  Derivative/1 -> Gain2/1
